simulink model "Failure_Detection"  (R2022b)
settings: Solver=FixedStepAuto  StartTime=0.0  StopTime=10.0  RelTol=1e-3
settings Model: Creator=MOHAMED  LastModifiedBy=عبدالرحيم
settings SolverCC: AlgebraicLoopSolver=TrustRegion
settings OptimizationCC: DefaultParameterBehavior=Inlined  UseDivisionForNetSlopeComputation=on  GainParamInheritBuiltInType=on  UseFloatMulNetSlope=on  InlineInvariantSignals=on  PassReuseOutputArgsAs=Individual arguments  ZeroExternalMemoryAtStartup=off  ZeroInternalMemoryAtStartup=off  NoFixptDivByZeroProtection=on  EfficientFloat2IntCast=on  LifeSpan=1  OptimizeBlockOrder=speed  DifferentSizesBufferReuse=on  EfficientTunableParamExpr=on
settings DebuggingCC: ParameterTunabilityLossMsg=error  SFMachineParentedDataDiag=warning  ArithmeticOperatorsInVariantConditions=warning
settings HardwareCC: ProdLongLongMode=on
settings SFSimCC: MATLABDynamicMemAlloc=off  CustomCodeUndefinedFunction=UseInterfaceOnly
settings RTWCC: Description=Embedded Coder  SystemTargetFile=ert.tlc  TemplateMakefile=ert_default_tmf
settings CodeAppCC: ForceParamTrailComments=on  IgnoreCustomStorageClasses=off  OperatorAnnotations=on  SimulinkDataObjDesc=on  SFDataObjDesc=on  CustomSymbolStrGlobalVar=rt$N$M  CustomSymbolStrType=$N$M  CustomSymbolStrFcn=$N$M$F  CustomSymbolStrMacro=$N$M  InsertBlockDesc=on
settings ERTTargetCC: TargetLangStandard=C99 (ISO)  GenerateSampleERTMain=on  IncludeMdlTerminateFcn=off  CombineSignalStateStructs=on  SupportAbsoluteTime=off  SupportComplex=off  SupportContinuousTime=on  InlinedParameterPlacement=NonHierarchical  ERTCustomFileTemplate=example_file_process.tlc  ERTFilePackagingFormat=CompactWithDataFile

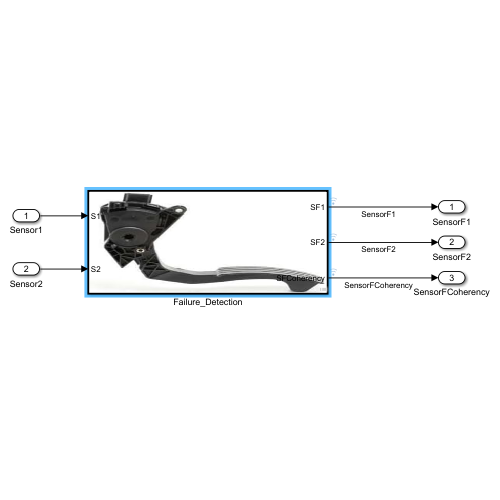
[thumbnail: Simulink's stored preview of the top-level diagram]
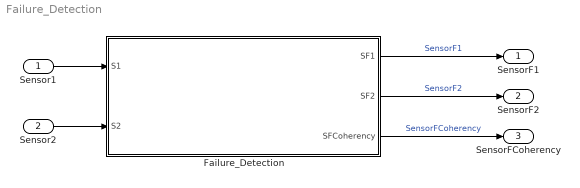
== system Failure_Detection ==
  Sensor1 : Inport
  Sensor2 : Inport  Port=2
  Failure_Detection : Subsystem  TreatAsAtomicUnit=on
      mask Display: image('WhatsApp Image 2025-03-08 at 23.21.02_ce8e83e1.jpg');
  SensorF1 : Outport
  SensorF2 : Outport  Port=2
  SensorFCoherency : Outport  Port=3
  wires:
  Sensor1/1 -> Failure_Detection/1(S1)
  Failure_Detection/3(SFCoherency) -> SensorFCoherency/1  "SensorFCoherency"
  Failure_Detection/2(SF2) -> SensorF2/1  "SensorF2"
  Failure_Detection/1(SF1) -> SensorF1/1  "SensorF1"
  Sensor2/1 -> Failure_Detection/2(S2)

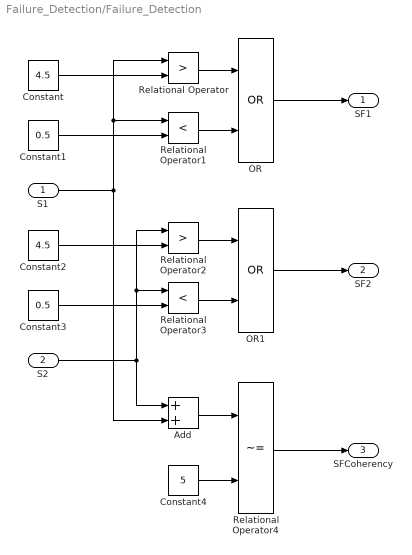
== system Failure_Detection/Failure_Detection ==
  S1 : Inport
  S2 : Inport  Port=2
  Add : Sum
  Constant : Constant  Value=4.5
  Constant1 : Constant  Value=0.5
  Constant2 : Constant  Value=4.5
  Constant3 : Constant  Value=0.5
  Constant4 : Constant  Value=5
  OR : Logic  Operator=OR  AllPortsSameDT=off  OutDataTypeStr=boolean
  OR1 : Logic  Operator=OR  AllPortsSameDT=off  OutDataTypeStr=boolean
  Relational Operator : RelationalOperator  Operator=>  OutDataTypeStr=boolean  RndMeth=Simplest  InputSameDT=off
  Relational Operator1 : RelationalOperator  Operator=<  OutDataTypeStr=boolean  RndMeth=Simplest  InputSameDT=off
  Relational Operator2 : RelationalOperator  Operator=>  OutDataTypeStr=boolean  RndMeth=Simplest  InputSameDT=off
  Relational Operator3 : RelationalOperator  Operator=<  OutDataTypeStr=boolean  RndMeth=Simplest  InputSameDT=off
  Relational Operator4 : RelationalOperator  Operator=~=  OutDataTypeStr=boolean  RndMeth=Simplest  InputSameDT=off
  SF1 : Outport
  SF2 : Outport  Port=2
  SFCoherency : Outport  Port=3
  wires:
  Relational Operator/1 -> OR/1
  Constant1/1 -> Relational Operator1/2
  Constant/1 -> Relational Operator/2
  S1/1 -> Add/2, Relational Operator1/1, Relational Operator/1
  S2/1 -> Add/1, Relational Operator3/1, Relational Operator2/1
  Constant3/1 -> Relational Operator3/2
  Relational Operator3/1 -> OR1/2
  Constant2/1 -> Relational Operator2/2
  OR/1 -> SF1/1
  Relational Operator1/1 -> OR/2
  Add/1 -> Relational Operator4/1
  Relational Operator4/1 -> SFCoherency/1
  Constant4/1 -> Relational Operator4/2
  Relational Operator2/1 -> OR1/1
  OR1/1 -> SF2/1
